simulink model "write16bits"  (R2018a)
settings: Solver=VariableStepAuto  StartTime=0.0  StopTime=10.0  RelTol=1e-3
libraries: simulink x16, mbd_s32k14_ec_toolbox x16
settings Model: Creator=domanico  LastModifiedBy=domanico

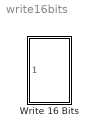
== system write16bits ==
  Write 16 Bits : Subsystem

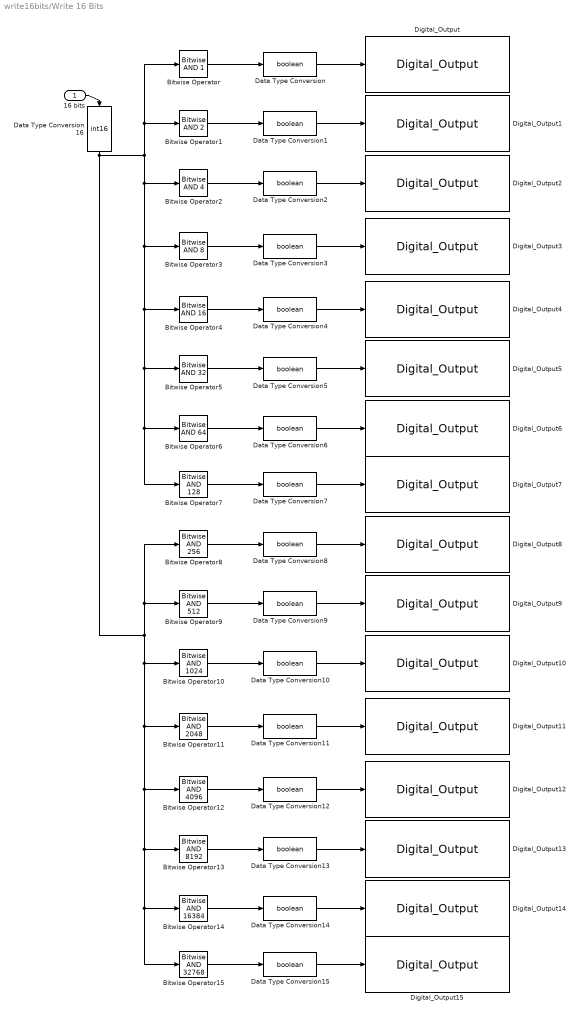
== system write16bits/Write 16 Bits ==
  16 bits : Inport
  Bitwise Operator : simulink/Logic and Bit Operations/Bitwise Operator  logicop=AND  UseBitMask=on  BitMask=1  BitMaskRealWorld=Stored Integer
  Bitwise Operator1 : simulink/Logic and Bit Operations/Bitwise Operator  logicop=AND  UseBitMask=on  BitMask=2  BitMaskRealWorld=Stored Integer
  Bitwise Operator10 : simulink/Logic and Bit Operations/Bitwise Operator  logicop=AND  UseBitMask=on  BitMask=1024  BitMaskRealWorld=Stored Integer
  Bitwise Operator11 : simulink/Logic and Bit Operations/Bitwise Operator  logicop=AND  UseBitMask=on  BitMask=2048  BitMaskRealWorld=Stored Integer
  Bitwise Operator12 : simulink/Logic and Bit Operations/Bitwise Operator  logicop=AND  UseBitMask=on  BitMask=4096  BitMaskRealWorld=Stored Integer
  Bitwise Operator13 : simulink/Logic and Bit Operations/Bitwise Operator  logicop=AND  UseBitMask=on  BitMask=8192  BitMaskRealWorld=Stored Integer
  Bitwise Operator14 : simulink/Logic and Bit Operations/Bitwise Operator  logicop=AND  UseBitMask=on  BitMask=16384  BitMaskRealWorld=Stored Integer
  Bitwise Operator15 : simulink/Logic and Bit Operations/Bitwise Operator  logicop=AND  UseBitMask=on  BitMask=32768  BitMaskRealWorld=Stored Integer
  Bitwise Operator2 : simulink/Logic and Bit Operations/Bitwise Operator  logicop=AND  UseBitMask=on  BitMask=4  BitMaskRealWorld=Stored Integer
  Bitwise Operator3 : simulink/Logic and Bit Operations/Bitwise Operator  logicop=AND  UseBitMask=on  BitMask=8  BitMaskRealWorld=Stored Integer
  Bitwise Operator4 : simulink/Logic and Bit Operations/Bitwise Operator  logicop=AND  UseBitMask=on  BitMask=16  BitMaskRealWorld=Stored Integer
  Bitwise Operator5 : simulink/Logic and Bit Operations/Bitwise Operator  logicop=AND  UseBitMask=on  BitMask=32  BitMaskRealWorld=Stored Integer
  Bitwise Operator6 : simulink/Logic and Bit Operations/Bitwise Operator  logicop=AND  UseBitMask=on  BitMask=64  BitMaskRealWorld=Stored Integer
  Bitwise Operator7 : simulink/Logic and Bit Operations/Bitwise Operator  logicop=AND  UseBitMask=on  BitMask=128  BitMaskRealWorld=Stored Integer
  Bitwise Operator8 : simulink/Logic and Bit Operations/Bitwise Operator  logicop=AND  UseBitMask=on  BitMask=256  BitMaskRealWorld=Stored Integer
  Bitwise Operator9 : simulink/Logic and Bit Operations/Bitwise Operator  logicop=AND  UseBitMask=on  BitMask=512  BitMaskRealWorld=Stored Integer
  Data Type Conversion{,1..15} (16 alike) : DataTypeConversion  OutDataTypeStr=boolean
  Data Type Conversion16 : DataTypeConversion  OutDataTypeStr=int16
  Digital_Output : mbd_s32k14_ec_toolbox/GPIO Blocks/Digital_Output  gpio_pin=PTD0: [PTD0 | Port D I/O]  drive_strength=Low
  Digital_Output1 : mbd_s32k14_ec_toolbox/GPIO Blocks/Digital_Output  gpio_pin=PTD1: [PTD1 | Port D I/O]  drive_strength=Low
  Digital_Output10 : mbd_s32k14_ec_toolbox/GPIO Blocks/Digital_Output  gpio_pin=PTD10: [PTD10 | Port D I/O]  drive_strength=Low
  Digital_Output11 : mbd_s32k14_ec_toolbox/GPIO Blocks/Digital_Output  gpio_pin=PTD11: [PTD11 | Port D I/O]  drive_strength=Low
  Digital_Output12 : mbd_s32k14_ec_toolbox/GPIO Blocks/Digital_Output  gpio_pin=PTD12: [PTD12 | Port D I/O]  drive_strength=Low
  Digital_Output13 : mbd_s32k14_ec_toolbox/GPIO Blocks/Digital_Output  gpio_pin=PTD13: [PTD13 | Port D I/O]  drive_strength=Low
  Digital_Output14 : mbd_s32k14_ec_toolbox/GPIO Blocks/Digital_Output  gpio_pin=PTD14: [PTD14 | Port D I/O]  drive_strength=Low
  Digital_Output15 : mbd_s32k14_ec_toolbox/GPIO Blocks/Digital_Output  gpio_pin=PTD15: [PTD15 | Port D I/O]  drive_strength=Low
  Digital_Output2 : mbd_s32k14_ec_toolbox/GPIO Blocks/Digital_Output  gpio_pin=PTD2: [PTD2 | Port D I/O]  drive_strength=Low
  Digital_Output3 : mbd_s32k14_ec_toolbox/GPIO Blocks/Digital_Output  gpio_pin=PTD3: [PTD3 | Port D I/O]  drive_strength=Low
  Digital_Output4 : mbd_s32k14_ec_toolbox/GPIO Blocks/Digital_Output  gpio_pin=PTD4: [PTD4 | Port D I/O]  drive_strength=Low
  Digital_Output5 : mbd_s32k14_ec_toolbox/GPIO Blocks/Digital_Output  gpio_pin=PTD5: [PTD5 | Port D I/O]  drive_strength=Low
  Digital_Output6 : mbd_s32k14_ec_toolbox/GPIO Blocks/Digital_Output  gpio_pin=PTD6: [PTD6 | Port D I/O]  drive_strength=Low
  Digital_Output7 : mbd_s32k14_ec_toolbox/GPIO Blocks/Digital_Output  gpio_pin=PTD7: [PTD7 | Port D I/O]  drive_strength=Low
  Digital_Output8 : mbd_s32k14_ec_toolbox/GPIO Blocks/Digital_Output  gpio_pin=PTD8: [PTD8 | Port D I/O]  drive_strength=Low
  Digital_Output9 : mbd_s32k14_ec_toolbox/GPIO Blocks/Digital_Output  gpio_pin=PTD9: [PTD9 | Port D I/O]  drive_strength=Low
  wires:
  Data Type Conversion4/1 -> Digital_Output4/1
  Data Type Conversion3/1 -> Digital_Output3/1
  Data Type Conversion2/1 -> Digital_Output2/1
  Data Type Conversion1/1 -> Digital_Output1/1
  Data Type Conversion/1 -> Digital_Output/1
  16 bits/1 -> Data Type Conversion16/1
  Bitwise Operator4/1 -> Data Type Conversion4/1
  Bitwise Operator3/1 -> Data Type Conversion3/1
  Bitwise Operator2/1 -> Data Type Conversion2/1
  Bitwise Operator1/1 -> Data Type Conversion1/1
  Bitwise Operator/1 -> Data Type Conversion/1
  Data Type Conversion5/1 -> Digital_Output5/1
  Bitwise Operator5/1 -> Data Type Conversion5/1
  Data Type Conversion6/1 -> Digital_Output6/1
  Bitwise Operator6/1 -> Data Type Conversion6/1
  Data Type Conversion7/1 -> Digital_Output7/1
  Bitwise Operator7/1 -> Data Type Conversion7/1
  Data Type Conversion12/1 -> Digital_Output12/1
  Data Type Conversion11/1 -> Digital_Output11/1
  Data Type Conversion10/1 -> Digital_Output10/1
  Data Type Conversion9/1 -> Digital_Output9/1
  Data Type Conversion8/1 -> Digital_Output8/1
  Bitwise Operator12/1 -> Data Type Conversion12/1
  Bitwise Operator11/1 -> Data Type Conversion11/1
  Bitwise Operator10/1 -> Data Type Conversion10/1
  Bitwise Operator9/1 -> Data Type Conversion9/1
  Bitwise Operator8/1 -> Data Type Conversion8/1
  Data Type Conversion13/1 -> Digital_Output13/1
  Bitwise Operator13/1 -> Data Type Conversion13/1
  Data Type Conversion14/1 -> Digital_Output14/1
  Bitwise Operator14/1 -> Data Type Conversion14/1
  Data Type Conversion15/1 -> Digital_Output15/1
  Bitwise Operator15/1 -> Data Type Conversion15/1
  Data Type Conversion16/1 -> Bitwise Operator2/1, Bitwise Operator3/1, Bitwise Operator4/1, Bitwise Operator5/1, Bitwise Operator6/1, Bitwise Operator7/1, Bitwise Operator1/1, Bitwise Operator/1, Bitwise Operator8/1, Bitwise Operator9/1, Bitwise Operator15/1, Bitwise Operator14/1, Bitwise Operator13/1, Bitwise Operator12/1, Bitwise Operator11/1, Bitwise Operator10/1
